simulink model "Target_Control_System"  (R2021b)
settings: Solver=FixedStepDiscrete  StartTime=0.0  StopTime=5  RelTol=1e-3
PreLoadFcn:
  | RTWConfigurationCB('preloadfcn', bdroot);
PostLoadFcn:
  | load('configuration/data_struct.mat');
  | load('configuration/fluxMaps_propMotor.mat');
  | load('configuration/parameterInit_PROP.mat');
  | load('configuration/parameterInit_PUMP.mat');
  | load('configuration/parameterInit_PITCH.mat');
  | load('configuration/parameterInit_TILT.mat');
  | %load('configuration/base_workspace_signal_definition.mat');
  | %load('resolvedatastores_to_baseworkspace_for_faster_simulation.mat');
model workspace (MAT data in the model file):
  SIMULATION_OPTIONS : Simulink.Parameter (value not decoded)
  TARGET_CODE_GEN : Simulink.Parameter (value not decoded)
  TCS_SAMPLE_FREQ_HZ : Simulink.Parameter (value not decoded)
symbols that are objects in the model workspace (value not decoded): TARGET_CODE_GEN, TCS_SAMPLE_FREQ_HZ
undefined symbols (not defined in the file): A_DQ_REF_LPF_INIT__PITCH, A_DQ_REF_LPF_INIT__PROP, A_DQ_REF_LPF_INIT__PUMP, A_DQ_REF_LPF_INIT__TILT, A_OBSERVER_CONFIDENCE_INIT__PITCH, A_OBSERVER_CONFIDENCE_INIT__PROP, A_OBSERVER_CONFIDENCE_INIT__PUMP, A_OBSERVER_CONFIDENCE_INIT__TILT, ACTUATOR_MAX_ANGLE_TRIP__PITCH, ACTUATOR_MIN_ANGLE_TRIP__PITCH, ACTUATOR_POS_SENSOR_INV_DIRECTION__PITCH, ACTUATOR_POS_SENSOR_INV_DIRECTION__TILT, ACTUATOR_POS_SENSOR_OFFSET__PITCH, ACTUATOR_POS_SENSOR_OFFSET__TILT, ADC_scaler1_baseaddr_TILT, ADC_SCALER_FLOAT_TO_FIXPOINT_EXPANSION, ANGLE_ELEC_FROM_SENSOR_OFFSET_INIT__PITCH, ANGLE_ELEC_FROM_SENSOR_OFFSET_INIT__PROP, ANGLE_ELEC_FROM_SENSOR_OFFSET_INIT__PUMP, ANGLE_ELEC_FROM_SENSOR_OFFSET_INIT__TILT, AUTO_CLEAR_FAULTS_ENABLED__PITCH, AUTO_CLEAR_FAULTS_ENABLED__PROP, AUTO_CLEAR_FAULTS_ENABLED__PUMP, AUTO_CLEAR_FAULTS_ENABLED__TILT, AUTO_CLEAR_FAULTS_WAIT_TICKS__PITCH, AUTO_CLEAR_FAULTS_WAIT_TICKS__PROP, AUTO_CLEAR_FAULTS_WAIT_TICKS__PUMP, AUTO_CLEAR_FAULTS_WAIT_TICKS__TILT, AUTO_I_ZERO_IDLE_TICKS__PITCH, AUTO_I_ZERO_IDLE_TICKS__PROP, AUTO_I_ZERO_IDLE_TICKS__PUMP, AUTO_I_ZERO_IDLE_TICKS__TILT, AUTO_I_ZERO_OFFSET_IDC_THRESHOLD__PITCH, AUTO_I_ZERO_OFFSET_IDC_THRESHOLD__PROP, AUTO_I_ZERO_OFFSET_IDC_THRESHOLD__PUMP, AUTO_I_ZERO_OFFSET_IDC_THRESHOLD__TILT, AUTO_I_ZERO_OFFSET_IPH_THRESHOLD__PITCH, AUTO_I_ZERO_OFFSET_IPH_THRESHOLD__PROP, AUTO_I_ZERO_OFFSET_IPH_THRESHOLD__PUMP, AUTO_I_ZERO_OFFSET_IPH_THRESHOLD__TILT, AUTO_SENSORLESS_SWITCHOVER_DISABLE_OMEGA, AUTO_SENSORLESS_SWITCHOVER_ENABLE_OMEGA, AUTO_SENSORLESS_SWITCHOVER_MIN_CONFIDENCE, AUXILIARY_PROTECTION_UNIT_BASEADDR__TILT, blanking_max_error_omega_INIT_PITCH, blanking_max_error_omega_INIT_TILT, blanking_max_error_position_INIT_PITCH, blanking_max_error_position_INIT_TILT, BRUTE_START_I_Q_REF_RAMP_SPEED__PITCH, BRUTE_START_I_Q_REF_RAMP_SPEED__PROP, BRUTE_START_I_Q_REF_RAMP_SPEED__PUMP, BRUTE_START_I_Q_REF_RAMP_SPEED__TILT, CONTROL_LOOP_DT_INIT__PITCH, CONTROL_LOOP_DT_INIT__PROP, CONTROL_LOOP_DT_INIT__PUMP, CONTROL_LOOP_DT_INIT__TILT, CORRECTION_FILTER_SCALE__PITCH, CORRECTION_FILTER_SCALE__PROP, CORRECTION_FILTER_SCALE__PUMP, CORRECTION_FILTER_SCALE__TILT ... (+458)
libraries: simulink x178, Reusables_Lib x24
(part 11 of 47)

== system Target_Control_System/Target_Control_System/InterruptFunction/propMotor_isrTask/currentController/Subsystem ==
  Enable : EnablePort
  Abs : Abs
  Abs1 : Abs
  Add1 : Sum
  Data Store Read10 : DataStoreRead  DataStoreName=oProp  DataStoreElements=oProp.oIsr_.oIn_.fFluxFeedforwardGainRampOut_  IndexOptions=Index vector (dialog)  Indices=1  OutputSizes=1
  Data Store Read11 : DataStoreRead  DataStoreName=oProp  DataStoreElements=oProp.oIsr_.oState_.fId_  IndexOptions=Index vector (dialog)  Indices=1  OutputSizes=1
  Data Store Read12 : DataStoreRead  DataStoreName=oProp  DataStoreElements=oProp.oIsr_.oParam_.oPiDataId_.oParameter_.fKp_  IndexOptions=Index vector (dialog)  Indices=1  OutputSizes=1
  Data Store Read13 : DataStoreRead  DataStoreName=oProp  DataStoreElements=oProp.oIsr_.oIn_.fOneOverUdc_  IndexOptions=Index vector (dialog)  Indices=1  OutputSizes=1
  Data Store Read14 : DataStoreRead  DataStoreName=oProp  DataStoreElements=oProp.oIsr_.oIn_.fOneOverUdc_  IndexOptions=Index vector (dialog)  Indices=1  OutputSizes=1
  Data Store Read15 : DataStoreRead  DataStoreName=mdl_prop_fOmegaE  IndexOptions=Index vector (dialog)  Indices=1  OutputSizes=1
  Data Store Read16 : DataStoreRead  DataStoreName=mdl_prop_fOmegaE  IndexOptions=Index vector (dialog)  Indices=1  OutputSizes=1
  Data Store Read17 : DataStoreRead  DataStoreName=oProp  DataStoreElements=oProp.oIsr_.oParam_.fOverspeedProtectionLimitOmegaE_  IndexOptions=Index vector (dialog)  Indices=1  OutputSizes=1
  Data Store Read18 : DataStoreRead  DataStoreName=oProp  DataStoreElements=oProp.oIsr_.oIn_.fIqRefRampOut_  IndexOptions=Index vector (dialog)  Indices=1  OutputSizes=1
  Data Store Read19 : DataStoreRead  DataStoreName=oProp  DataStoreElements=oProp.oIsr_.oState_.fSoftILimitActual_  IndexOptions=Index vector (dialog)  Indices=1  OutputSizes=1
  Data Store Read2 : DataStoreRead  DataStoreName=oProp  DataStoreElements=oProp.oIsr_.oState_.fIq_  IndexOptions=Index vector (dialog)  Indices=1  OutputSizes=1
  Data Store Read24 : DataStoreRead  DataStoreName=oProp  DataStoreElements=oProp.oIsr_.oParam_.oPiDataId_.oParameter_.fLoopDt_  IndexOptions=Index vector (dialog)  Indices=1  OutputSizes=1
  Data Store Read25 : DataStoreRead  DataStoreName=oProp  DataStoreElements=oProp.oIsr_.oParam_.oPiDataId_.oParameter_.fIntMax_  IndexOptions=Index vector (dialog)  Indices=1  OutputSizes=1
  Data Store Read26 : DataStoreRead  DataStoreName=oProp  DataStoreElements=oProp.oIsr_.oParam_.oPiDataId_.oParameter_.fOutMax_  IndexOptions=Index vector (dialog)  Indices=1  OutputSizes=1
  Data Store Read27 : DataStoreRead  DataStoreName=oProp  DataStoreElements=oProp.oIsr_.oParam_.fMaximumVoltageVectorLengthSquared_  IndexOptions=Index vector (dialog)  Indices=1  OutputSizes=1
  Data Store Read28 : DataStoreRead  DataStoreName=oProp  DataStoreElements=oProp.oIsr_.oParam_.oPiDataId_.oParameter_.fIntMin_  IndexOptions=Index vector (dialog)  Indices=1  OutputSizes=1
  Data Store Read29 : DataStoreRead  DataStoreName=oProp  DataStoreElements=oProp.oIsr_.oParam_.oPiDataId_.oParameter_.fOutMin_  IndexOptions=Index vector (dialog)  Indices=1  OutputSizes=1
  Data Store Read3 : DataStoreRead  DataStoreName=oProp  DataStoreElements=oProp.oIsr_.oIn_.fIdRefFractionOfIq_  IndexOptions=Index vector (dialog)  Indices=1  OutputSizes=1
  Data Store Read30 : DataStoreRead  DataStoreName=oProp  DataStoreElements=oProp.oIsr_.oParam_.oPiDataIq_.oParameter_.fKp_  IndexOptions=Index vector (dialog)  Indices=1  OutputSizes=1
  Data Store Read33 : DataStoreRead  DataStoreName=oProp  DataStoreElements=oProp.oIsr_.oParam_.oPiDataIq_.oParameter_.fLoopDt_  IndexOptions=Index vector (dialog)  Indices=1  OutputSizes=1
  Data Store Read34 : DataStoreRead  DataStoreName=oProp  DataStoreElements=oProp.oIsr_.oParam_.oPiDataIq_.oParameter_.fIntMax_  IndexOptions=Index vector (dialog)  Indices=1  OutputSizes=1
  Data Store Read35 : DataStoreRead  DataStoreName=oProp  DataStoreElements=oProp.oIsr_.oParam_.oPiDataIq_.oParameter_.fOutMax_  IndexOptions=Index vector (dialog)  Indices=1  OutputSizes=1
  Data Store Read36 : DataStoreRead  DataStoreName=oProp  DataStoreElements=oProp.oIsr_.oParam_.oPiDataIq_.oParameter_.fIntMin_  IndexOptions=Index vector (dialog)  Indices=1  OutputSizes=1
  Data Store Read37 : DataStoreRead  DataStoreName=oProp  DataStoreElements=oProp.oIsr_.oParam_.oPiDataIq_.oParameter_.fOutMin_  IndexOptions=Index vector (dialog)  Indices=1  OutputSizes=1
  Data Store Read4 : DataStoreRead  DataStoreName=oProp  DataStoreElements=oProp.oIsr_.oIn_.fIdRefRampOut_  IndexOptions=Index vector (dialog)  Indices=1  OutputSizes=1
  Data Store Read40 : DataStoreRead  DataStoreName=oProp  DataStoreElements=oProp.oIsr_.oParam_.oPiDataIq_.oParameter_.fKi_  IndexOptions=Index vector (dialog)  Indices=1  OutputSizes=1
  Data Store Read5 : DataStoreRead  DataStoreName=oProp  DataStoreElements=oProp.oIsr_.oParam_.oPiDataId_.fState_  IndexOptions=Index vector (dialog)  Indices=1  OutputSizes=1
  Data Store Read6 : DataStoreRead  DataStoreName=oProp  DataStoreElements=oProp.oIsr_.oIn_.fOneOverUdc_  IndexOptions=Index vector (dialog)  Indices=1  OutputSizes=1
  Data Store Read7 : DataStoreRead  DataStoreName=oProp  DataStoreElements=oProp.oIsr_.oParam_.oPiDataId_.oParameter_.fKi_  IndexOptions=Index vector (dialog)  Indices=1  OutputSizes=1
  Data Store Read8 : DataStoreRead  DataStoreName=oProp  DataStoreElements=oProp.oIsr_.oParam_.oPiDataIq_.fState_  IndexOptions=Index vector (dialog)  Indices=1  OutputSizes=1
  Data Store Read9 : DataStoreRead  DataStoreName=oProp  DataStoreElements=oProp.oIsr_.oState_.fFluxMainMagnitudeLpf_  IndexOptions=Index vector (dialog)  Indices=1  OutputSizes=1
  Data Store Write1 : DataStoreWrite  DataStoreName=oProp  DataStoreElements=oProp.oIsr_.oState_.fUqRefPiContrib_  IndexOptions=Index vector (dialog)  Indices=1  OutputSizes=1
  Data Store Write2 : DataStoreWrite  DataStoreName=oProp  DataStoreElements=oProp.oIsr_.oState_.fUdRef_  IndexOptions=Index vector (dialog)  Indices=1  OutputSizes=1
  Data Store Write3 : DataStoreWrite  DataStoreName=oProp  DataStoreElements=oProp.oIsr_.oState_.fUqRef_  IndexOptions=Index vector (dialog)  Indices=1  OutputSizes=1
  Data Store Write31 : DataStoreWrite  DataStoreName=oProp  DataStoreElements=oProp.oIsr_.oParam_.oPiDataId_.fState_  IndexOptions=Index vector (dialog)  Indices=1  OutputSizes=1
  Data Store Write8 : DataStoreWrite  DataStoreName=oProp  DataStoreElements=oProp.oIsr_.oParam_.oPiDataIq_.fState_  IndexOptions=Index vector (dialog)  Indices=1  OutputSizes=1
  Divide1 : Product  Inputs=**
  Equal : RelationalOperator  Operator=>  OutDataTypeStr=boolean  RndMeth=Simplest
  Equal3 : RelationalOperator  Operator=<  OutDataTypeStr=boolean  RndMeth=Simplest
  Flux Feed-forward : Subsystem
  Limit Voltage Vector : Subsystem
  NOT : Logic  Operator=NOT  AllPortsSameDT=off  OutDataTypeStr=boolean
  PI Id Current Controller : Subsystem
  PI Iq Current Controller : Subsystem
  Product : Product
  Product1 : Product
  Sign : Signum
  Subsystem : Subsystem
  Subsystem1 : Subsystem
  Switch : Switch  Criteria=u2 > Threshold
  Switch1 : Switch  Criteria=u2 > Threshold
  wires:
  Subsystem1/1(Output) -> Switch1/3
  Subsystem/1(Output) -> Switch1/1
  Switch1/1 -> Product1/2  "fOverspeedProtectionScaler_"
  Switch/1 -> Product1/1  "fTemp"
  Sign/1 -> Product/1
  Product/1 -> Switch/1
  Equal3/1 -> Switch/2
  Data Store Read19/1 -> Equal3/1, Product/2
  Abs1/1 -> Equal3/2
  Data Store Read18/1 -> Abs1/1, Switch/3, Sign/1
  NOT/1 -> Subsystem1/Enable
  Equal/1 -> Subsystem/Enable, NOT/1, Switch1/2
  Data Store Read17/1 -> Equal/2
  Abs/1 -> Equal/1
  Data Store Read15/1 -> Abs/1
  Add1/1 -> PI Id Current Controller/2(fTarget)
  Data Store Read4/1 -> Add1/1
  Data Store Read10/1 -> Flux Feed-forward/3(fFluxFeedforwardGainRampOut)
  Divide1/1 -> Add1/2
  Data Store Read13/1 -> Flux Feed-forward/4(fOneOverUdc)
  Flux Feed-forward/1(fUqRef) -> Limit Voltage Vector/3(fUqRef)
  Data Store Read27/1 -> Limit Voltage Vector/2(fMaximumVoltageVectorLengthSquared)
  Data Store Read16/1 -> Flux Feed-forward/5(mdl_tilt_fOmegaE)
  Limit Voltage Vector/1(fUdRef_out) -> Data Store Write2/1
  PI Id Current Controller/1(fOutput) -> Limit Voltage Vector/1(fUdRef)
  Data Store Read3/1 -> Divide1/1
  Product1/1 -> PI Iq Current Controller/2(fTarget), Divide1/2
  Data Store Read9/1 -> Flux Feed-forward/2(fFluxMainMagnitudeLpf)
  Limit Voltage Vector/2(fUqRef_out) -> Data Store Write3/1
  PI Iq Current Controller/1(fOutput) -> Flux Feed-forward/1(fUqRefPiContrib), Data Store Write1/1
  Data Store Read36/1 -> PI Iq Current Controller/9(fIntMin)
  PI Id Current Controller/2(*fpState) -> Data Store Write31/1
  Data Store Read34/1 -> PI Iq Current Controller/7(fIntMax)
  Data Store Read8/1 -> PI Iq Current Controller/11(fState)
  Data Store Read12/1 -> PI Id Current Controller/3(fKp)
  Data Store Read26/1 -> PI Id Current Controller/8(fOutMax)
  Data Store Read40/1 -> PI Iq Current Controller/4(fKi)
  PI Iq Current Controller/2(*fpState) -> Data Store Write8/1
  Data Store Read35/1 -> PI Iq Current Controller/8(fOutMax)
  Data Store Read14/1 -> PI Id Current Controller/5(fScale)
  Data Store Read30/1 -> PI Iq Current Controller/3(fKp)
  Data Store Read5/1 -> PI Id Current Controller/11(fState)
  Data Store Read37/1 -> PI Iq Current Controller/10(fOutMin)
  Data Store Read7/1 -> PI Id Current Controller/4(fKi)
  Data Store Read2/1 -> PI Iq Current Controller/1(fActual)
  Data Store Read33/1 -> PI Iq Current Controller/6(fLoopDt)
  Data Store Read6/1 -> PI Iq Current Controller/5(fScale)
  Data Store Read11/1 -> PI Id Current Controller/1(fActual)
  Data Store Read29/1 -> PI Id Current Controller/10(fOutMin)
  Data Store Read24/1 -> PI Id Current Controller/6(fLoopDt)
  Data Store Read25/1 -> PI Id Current Controller/7(fIntMax)
  Data Store Read28/1 -> PI Id Current Controller/9(fIntMin)

== system Target_Control_System/Target_Control_System/InterruptFunction/propMotor_isrTask/fluxAngleCalculation/Angle Clip ==
  Angle_In : Inport
  Add1 : Sum  Inputs=-+
  Add12 : Sum  Inputs=-+
  Add2 : Sum
  Add3 : Sum
  Equal1 : RelationalOperator  Operator=>  OutDataTypeStr=boolean  RndMeth=Simplest
  Equal2 : RelationalOperator  Operator=<  OutDataTypeStr=boolean  RndMeth=Simplest
  Equal3 : RelationalOperator  Operator=<  OutDataTypeStr=boolean  RndMeth=Simplest
  Equal5 : RelationalOperator  Operator=>  OutDataTypeStr=boolean  RndMeth=Simplest
  Pi : Constant  Value=pi  OutDataTypeStr=single  SampleTime=-1
  Pi1 : Constant  Value=2*pi  OutDataTypeStr=single  SampleTime=-1
  Pi2 : Constant  Value=-pi  OutDataTypeStr=single  SampleTime=-1
  Pi3 : Constant  Value=2*pi  OutDataTypeStr=single  SampleTime=-1
  Pi4 : Constant  Value=-pi  OutDataTypeStr=single  SampleTime=-1
  Pi8 : Constant  Value=pi  OutDataTypeStr=single  SampleTime=-1
  Switch{1..3,5} (4 alike) : Switch  Criteria=u2 > Threshold  Threshold=0.5
  Angle_Out : Outport
  wires:
  Switch3/1 -> Switch2/1
  Equal2/1 -> Switch3/2
  Switch5/1 -> Switch2/3, Add3/2, Equal3/1
  Add2/1 -> Switch3/1
  Pi3/1 -> Add3/1, Add2/1
  Add3/1 -> Switch3/3, Equal2/1, Add2/2
  Pi4/1 -> Equal2/2
  Switch2/1 -> Angle_Out/1
  Equal3/1 -> Switch2/2
  Pi2/1 -> Equal3/2
  Switch1/1 -> Switch5/1
  Add1/1 -> Switch1/1
  Equal5/1 -> Switch1/2
  Pi8/1 -> Equal5/2
  Add12/1 -> Equal5/1, Add1/2, Switch1/3
  Pi/1 -> Equal1/2
  Equal1/1 -> Switch5/2
  Angle_In/1 -> Add12/2, Equal1/1, Switch5/3
  Pi1/1 -> Add12/1, Add1/1

== system Target_Control_System/Target_Control_System/InterruptFunction/propMotor_isrTask/fluxAngleCalculation/ModelSource ==
  note: 1) Add Subsystem or Model blocks as valid variant choices.
      | 2) You cannot connect blocks at this level. At simulation, connectivity is automatically
      | determined, based on the active variant and port name matching.
  DoNotIncludeCustomCode : Subsystem  TreatAsAtomicUnit=on  VariantControl=TARGET_CODE_GEN == 0
  IncludeCustomCode : Subsystem  TreatAsAtomicUnit=on  VariantControl=(default)

== system Target_Control_System/Target_Control_System/InterruptFunction/propMotor_isrTask/fluxAngleCalculation/Subsystem ==
  Enable : EnablePort
  Data Store Read66 : DataStoreRead  DataStoreName=oProp  DataStoreElements=oProp.oIsr_.oIn_.fOmegaERefRampOut_  IndexOptions=Index vector (dialog)  Indices=1  OutputSizes=1
  Integrator with Angle Wrapper : Subsystem
  Integrator with Angle Wrapper_OLD : Subsystem  Commented=on
  Angle : Outport
  wires:
  Integrator with Angle Wrapper/1(Angle) -> Angle/1
  Data Store Read66/1 -> Integrator with Angle Wrapper/1(Omega)

== system Target_Control_System/Target_Control_System/InterruptFunction/propMotor_isrTask/fluxAngleCalculation/Subsystem1 ==
  In1 : Inport
  In2 : Inport  Port=2
  Enable : EnablePort
  Add1 : Sum
  Angle Clip : Subsystem
  Angle_Out : Outport
  wires:
  Add1/1 -> Angle Clip/1(Angle_In)
  In2/1 -> Add1/2
  In1/1 -> Add1/1
  Angle Clip/1(Angle_Out) -> Angle_Out/1

== system Target_Control_System/Target_Control_System/InterruptFunction/propMotor_isrTask/fluxAngleCalculation/vsincos()1 ==
  fFluxMasterAngle : Inport
  fFluxMasterAngleBdwd : Inport  Port=2
  Enable : EnablePort
  Cos2 : Trigonometry  Operator=cos
  Cos3 : Trigonometry  Operator=cos
  Data Store Write1 : DataStoreWrite  DataStoreName=mdl_fFluxMasterAngle_cos_  IndexOptions=Index vector (dialog)  Indices=1  OutputSizes=1
  Data Store Write2 : DataStoreWrite  DataStoreName=mdl_fFluxMasterAngle_sin_  IndexOptions=Index vector (dialog)  Indices=1  OutputSizes=1
  Data Store Write7 : DataStoreWrite  DataStoreName=mdl_fFluxMasterAngleBkwd_sin_  IndexOptions=Index vector (dialog)  Indices=1  OutputSizes=1
  Data Store Write8 : DataStoreWrite  DataStoreName=mdl_fFluxMasterAngleBkwd_cos_  IndexOptions=Index vector (dialog)  Indices=1  OutputSizes=1
  Sin2 : Trigonometry
  Sin3 : Trigonometry
  wires:
  fFluxMasterAngle/1 -> Sin2/1, Cos2/1
  fFluxMasterAngleBdwd/1 -> Sin3/1, Cos3/1
  Sin2/1 -> Data Store Write2/1
  Cos2/1 -> Data Store Write1/1
  Sin3/1 -> Data Store Write7/1
  Cos3/1 -> Data Store Write8/1

== system Target_Control_System/Target_Control_System/InterruptFunction/propMotor_isrTask/fluxObserver/piControllerStep_fOmegaE1 ==
  fActual : Inport
  fTarget : Inport  Port=2
  fKp : Inport  Port=3
  fKi : Inport  Port=4
  fScale : Inport  Port=5
  fLoopDt : Inport  Port=6
  fIntMax : Inport  Port=7
  fOutMax : Inport  Port=8
  fIntMin : Inport  Port=9
  fOutMin : Inport  Port=10
  fState : Inport  Port=11
  Add : Sum  Inputs=|++
  Mux : Mux  Inputs=3
  Mux1 : Mux  Inputs=3
  Product : Product
  Saturation Dynamic : simulink/Discontinuities/Saturation Dynamic  OutMin=[]  OutMax=[]  OutDataTypeStr=Inherit: Same as second input  OutDataType=fixdt(1, 16)  OutScaling=2^-10  DoSatur=off
  Saturation Dynamic1 : simulink/Discontinuities/Saturation Dynamic  OutMin=[]  OutMax=[]  OutDataTypeStr=Inherit: Same as second input  OutDataType=fixdt(1, 16)  OutScaling=2^-10  DoSatur=off
  Scope3 : Scope  NumInputPorts=6
  Sum1 : Sum  Inputs=++|
  Sum22 : Sum  Inputs=-+|
  fError * fKi_ * fScale : Fcn  Expr=u(1)*u(2)*u(3)
  fError * fKp_ * fScale1 : Fcn  Expr=u(1)*u(2)*u(3)
  fOutput : Outport
  *fpState : Outport  Port=2
  wires:
  fLoopDt/1 -> Product/2
  fOutMax/1 -> Saturation Dynamic1/1
  fOutMin/1 -> Saturation Dynamic1/3
  fIntMin/1 -> Saturation Dynamic/3
  fIntMax/1 -> Saturation Dynamic/1
  Add/1 -> Saturation Dynamic/2
  fState/1 -> Add/2
  Product/1 -> Add/1
  Mux1/1 -> fError * fKp_ * fScale1/1
  fKi/1 -> Mux/2
  fScale/1 -> Mux/1, Mux1/3
  fKp/1 -> Mux1/2
  Mux/1 -> fError * fKi_ * fScale/1
  Saturation Dynamic1/1 -> fOutput/1, Scope3/6
  Sum1/1 -> Saturation Dynamic1/2  "fError"
  fError * fKp_ * fScale1/1 -> Sum1/1, Scope3/4
  Saturation Dynamic/1 -> Scope3/5, *fpState/1, Sum1/2  "*fpState"
  fActual/1 -> Sum22/1, Scope3/2
  fTarget/1 -> Sum22/2, Scope3/1
  fError * fKi_ * fScale/1 -> Product/1
  Sum22/1 -> Scope3/3, Mux/3, Mux1/1  "fError"

== system Target_Control_System/Target_Control_System/InterruptFunction/propMotor_isrTask/pwmGeneration/Subsystem ==
  note: // moved here, originating from main layer
      | // Ramp soft current limit back up to the setpoint (it is reduced in the main interrupt loop)
  Enable : EnablePort
  Constant1 : Constant  OutDataTypeStr=int32  SampleTime=-1
  Constant11 : Constant  Value=-1  SampleTime=-1
  Constant12 : Constant  Value=-1  SampleTime=-1
  Constant13 : Constant  Value=-1  SampleTime=-1
  Constant2 : Constant  Value=0.5  OutDataTypeStr=single  SampleTime=-1
  Constant4 : Constant  Value=0.5  OutDataTypeStr=single  SampleTime=-1
  Constant6 : Constant  Value=0.5  OutDataTypeStr=single  SampleTime=-1
  Data Store Read1 : DataStoreRead  DataStoreName=mdl_fFluxMasterAngleBkwd_cos_  IndexOptions=Index vector (dialog)  Indices=1  OutputSizes=1
  Data Store Read10 : DataStoreRead  DataStoreName=oProp  DataStoreElements=oProp.oIsr_.oParam_.fMaximumDuty_  IndexOptions=Index vector (dialog)  Indices=1  OutputSizes=1
  Data Store Read11 : DataStoreRead  DataStoreName=oProp  DataStoreElements=oProp.oIsr_.oParam_.fMaximumDuty_  IndexOptions=Index vector (dialog)  Indices=1  OutputSizes=1
  Data Store Read12 : DataStoreRead  DataStoreName=oProp  DataStoreElements=oProp.oIsr_.oState_.fSoftILimitActual_  IndexOptions=Index vector (dialog)  Indices=1  OutputSizes=1
  Data Store Read13 : DataStoreRead  DataStoreName=mdl_fFluxMasterAngleBkwd_sin_  IndexOptions=Index vector (dialog)  Indices=1  OutputSizes=1
  Data Store Read14 : DataStoreRead  DataStoreName=oProp  DataStoreElements=oProp.oIsr_.oParam_.fSoftILimitA_  IndexOptions=Index vector (dialog)  Indices=1  OutputSizes=1
  Data Store Read18 : DataStoreRead  DataStoreName=oProp  DataStoreElements=oProp.oIsr_.oParam_.fHalfPositiveDuty_  IndexOptions=Index vector (dialog)  Indices=1  OutputSizes=1
  Data Store Read19 : DataStoreRead  DataStoreName=oProp  DataStoreElements=oProp.oIsr_.oParam_.iInverseDirection_  IndexOptions=Index vector (dialog)  Indices=1  OutputSizes=1
  Data Store Read2 : DataStoreRead  DataStoreName=oProp  DataStoreElements=oProp.oIsr_.oState_.fUdRef_  IndexOptions=Index vector (dialog)  Indices=1  OutputSizes=1
  Data Store Read3 : DataStoreRead  DataStoreName=oProp  DataStoreElements=oProp.oIsr_.oState_.fUqRef_  IndexOptions=Index vector (dialog)  Indices=1  OutputSizes=1
  Data Store Read4 : DataStoreRead  DataStoreName=oProp  DataStoreElements=oProp.oIsr_.oParam_.fHalfPositiveDuty_  IndexOptions=Index vector (dialog)  Indices=1  OutputSizes=1
  Data Store Read5 : DataStoreRead  DataStoreName=oProp  DataStoreElements=oProp.oIsr_.oParam_.fHalfPositiveDuty_  IndexOptions=Index vector (dialog)  Indices=1  OutputSizes=1
  Data Store Read6 : DataStoreRead  DataStoreName=oProp  DataStoreElements=oProp.oIsr_.oParam_.fPwmPeriodTicksFloat_  IndexOptions=Index vector (dialog)  Indices=1  OutputSizes=1
  Data Store Read7 : DataStoreRead  DataStoreName=oProp  DataStoreElements=oProp.oIsr_.oParam_.fPwmPeriodTicksFloat_  IndexOptions=Index vector (dialog)  Indices=1  OutputSizes=1
  Data Store Read8 : DataStoreRead  DataStoreName=oProp  DataStoreElements=oProp.oIsr_.oParam_.fPwmPeriodTicksFloat_  IndexOptions=Index vector (dialog)  Indices=1  OutputSizes=1
  Data Store Read9 : DataStoreRead  DataStoreName=oProp  DataStoreElements=oProp.oIsr_.oParam_.fMaximumDuty_  IndexOptions=Index vector (dialog)  Indices=1  OutputSizes=1
  Data Store Write2 : DataStoreWrite  DataStoreName=oProp  DataStoreElements=oProp.oIsr_.oOut_.uiPwmDutyTicksB_  IndexOptions=Index vector (dialog)  Indices=1  OutputSizes=1
  Data Store Write27 : DataStoreWrite  DataStoreName=oProp  DataStoreElements=oProp.oIsr_.oState_.iPwmUpdated_  IndexOptions=Index vector (dialog)  Indices=1  OutputSizes=1
  Data Store Write3 : DataStoreWrite  DataStoreName=oProp  DataStoreElements=oProp.oIsr_.oOut_.uiPwmDutyTicksC_  IndexOptions=Index vector (dialog)  Indices=1  OutputSizes=1
  Data Store Write5 : DataStoreWrite  DataStoreName=oProp  DataStoreElements=oProp.oIsr_.oOut_.uiPwmDutyTicksA_  IndexOptions=Index vector (dialog)  Indices=1  OutputSizes=1
  Data Type Conversion : DataTypeConversion  OutDataTypeStr=uint32
  Data Type Conversion1 : DataTypeConversion  OutDataTypeStr=uint32
  Data Type Conversion2 : DataTypeConversion  OutDataTypeStr=uint32
  Demux : Demux  Outputs=3
  Equal : RelationalOperator  Operator=~=  OutDataTypeStr=boolean  RndMeth=Simplest
  Gain4 : Gain  Gain=0.5
  Max : MinMax  Function=max  Inputs=3
  Max1 : MinMax  Inputs=3
  Mux : Mux  Inputs=2
  Mux5 : Mux
  Product{1,6..10} (6 alike) : Product
  Saturation Dynamic : simulink/Discontinuities/Saturation Dynamic  OutMin=[]  OutMax=[]  OutDataTypeStr=Inherit: Same as second input  OutDataType=fixdt(1, 16)  OutScaling=2^-10  DoSatur=off
  Saturation Dynamic1 : simulink/Discontinuities/Saturation Dynamic  OutMin=[]  OutMax=[]  OutDataTypeStr=Inherit: Same as second input  OutDataType=fixdt(1, 16)  OutScaling=2^-10  DoSatur=off
  Saturation Dynamic2 : simulink/Discontinuities/Saturation Dynamic  OutMin=[]  OutMax=[]  OutDataTypeStr=Inherit: Same as second input  OutDataType=fixdt(1, 16)  OutScaling=2^-10  DoSatur=off
  Subsystem : Subsystem
  Sum1 : Sum  Inputs=|++  OutDataTypeStr=single
  Sum4 : Sum  Inputs=|++  OutDataTypeStr=single
  Sum5 : Sum  Inputs=|++  OutDataTypeStr=single
  Sum6 : Sum  OutDataTypeStr=single
  Sum7 : Sum  Inputs=|+-  OutDataTypeStr=single
  Sum8 : Sum  Inputs=|+-  OutDataTypeStr=single
  Sum9 : Sum  Inputs=|+-  OutDataTypeStr=single
  Switch1 : Switch  Criteria=u2 > Threshold
  alpha/beta to abc1 : Gain  Gain="[1  0; -0.5 sqrt(3)/2; -0.5 -sqrt(3)/2]"  Multiplication=Matrix(K*u) (u vector)
  alpha/beta to abc_inverseDirection1 : Gain  Gain="[1  0; -0.5 -sqrt(3)/2; -0.5 sqrt(3)/2]"  Multiplication=Matrix(K*u) (u vector)
  fUAlphaRef_ = afOutArray[3]*fUdRef - afOutArray[2]*fUqRef : Fcn  Expr=u(4)*u(1)-u(3)*u(2)
  fUBetaRef_ = afOutArray[3]*fUqRef + afOutArray[2]*fUdRef : Fcn  Expr=u(4)*u(2)+u(3)*u(1)
  wires:
  Constant1/1 -> Data Store Write27/1
  Equal/1 -> Subsystem/Enable
  Data Store Read14/1 -> Equal/2
  Data Store Read12/1 -> Equal/1
  alpha/beta to abc_inverseDirection1/1 -> Switch1/1
  Demux/3 -> Sum9/1, Max1/3, Max/3
  Data Store Read9/1 -> Saturation Dynamic/1
  Constant4/1 -> Sum4/2
  Mux5/1 -> fUAlphaRef_ = afOutArray[3]*fUdRef - afOutArray[2]*fUqRef/1, fUBetaRef_ = afOutArray[3]*fUqRef + afOutArray[2]*fUdRef/1
  Data Store Read8/1 -> Product10/2
  Sum6/1 -> Gain4/1  "Umax+Umin"
  Product1/1 -> Sum1/1
  Data Type Conversion/1 -> Data Store Write5/1
  Constant2/1 -> Sum1/2
  Constant6/1 -> Sum5/2
  Data Store Read2/1 -> Mux5/1
  Data Store Read13/1 -> Mux5/3
  Gain4/1 -> Sum9/2, Sum7/2, Sum8/2
  Sum5/1 -> Product10/1
  Sum4/1 -> Product9/1
  Product8/1 -> Data Type Conversion/1
  Data Store Read3/1 -> Mux5/2
  Product10/1 -> Data Type Conversion2/1
  Saturation Dynamic1/1 -> Product6/1
  Mux/1 -> alpha/beta to abc_inverseDirection1/1, alpha/beta to abc1/1
  alpha/beta to abc1/1 -> Switch1/3
  Data Store Read6/1 -> Product8/2
  Demux/1 -> Max1/2, Max/1, Sum7/1
  Max/1 -> Sum6/1
  Constant11/1 -> Saturation Dynamic/3
  Sum7/1 -> Saturation Dynamic/2  "fUaRef"
  Sum8/1 -> Saturation Dynamic1/2  "fUbRef"
  Data Store Read7/1 -> Product9/2
  Data Store Read18/1 -> Product1/2
  Max1/1 -> Sum6/2
  Data Store Read5/1 -> Product7/2
  Product6/1 -> Sum4/1
  Saturation Dynamic/1 -> Product1/1
  Product9/1 -> Data Type Conversion1/1
  Data Store Read4/1 -> Product6/2
  Data Type Conversion2/1 -> Data Store Write3/1
  Demux/2 -> Max1/1, Max/2, Sum8/1
  Data Type Conversion1/1 -> Data Store Write2/1
  Sum1/1 -> Product8/1
  Sum9/1 -> Saturation Dynamic2/2  "fUcRef"
  Constant13/1 -> Saturation Dynamic2/3
  Data Store Read11/1 -> Saturation Dynamic2/1
  Switch1/1 -> Demux/1
  Data Store Read1/1 -> Mux5/4
  fUAlphaRef_ = afOutArray[3]*fUdRef - afOutArray[2]*fUqRef/1 -> Mux/1  "fUAlphaRef_"
  Constant12/1 -> Saturation Dynamic1/3
  Data Store Read19/1 -> Switch1/2
  Saturation Dynamic2/1 -> Product7/1
  fUBetaRef_ = afOutArray[3]*fUqRef + afOutArray[2]*fUdRef/1 -> Mux/2  "fUBetaRef_"
  Data Store Read10/1 -> Saturation Dynamic1/1
  Product7/1 -> Sum5/1

== system Target_Control_System/Target_Control_System/InterruptFunction/propMotor_isrTask/softCurrentLimiting/Subsystem ==
  note: // Some current exceeds the soft current limiter
  fMaxOvershoot : Inport
  Enable : EnablePort
  Abs : Abs
  Add : Sum  Inputs=-+
  Add1 : Sum  Inputs=+-
  Constant : Constant  Value=0  OutDataTypeStr=single  SampleTime=-1
  Constant1 : Constant  Value=0  OutDataTypeStr=single  SampleTime=-1
  Data Store Read1 : DataStoreRead  DataStoreName=oProp  DataStoreElements=oProp.oIsr_.oParam_.fSoftILimitKp_  IndexOptions=Index vector (dialog)  Indices=1  OutputSizes=1
  Data Store Read7 : DataStoreRead  DataStoreName=oProp  DataStoreElements=oProp.oIsr_.oIn_.fIqRefRampOut_  IndexOptions=Index vector (dialog)  Indices=1  OutputSizes=1
  Data Store Read8 : DataStoreRead  DataStoreName=oProp  DataStoreElements=oProp.oIsr_.oState_.fSoftILimitActual_  IndexOptions=Index vector (dialog)  Indices=1  OutputSizes=1
  Data Store Write10 : DataStoreWrite  DataStoreName=oProp  DataStoreElements=oProp.oIsr_.oState_.fSoftILimitActual_  IndexOptions=Index vector (dialog)  Indices=1  OutputSizes=1
  Equal1 : RelationalOperator  Operator=<  OutDataTypeStr=boolean  RndMeth=Simplest
  Equal3 : RelationalOperator  Operator=<  OutDataTypeStr=boolean  RndMeth=Simplest
  Product : Product
  Switch : Switch  Criteria=u2 > Threshold
  Switch1 : Switch  Criteria=u2 > Threshold
  wires:
  Constant1/1 -> Switch1/1
  Switch1/1 -> Data Store Write10/1
  Equal1/1 -> Switch1/2
  Constant/1 -> Equal1/2
  Add1/1 -> Switch/3
  Data Store Read1/1 -> Product/1
  fMaxOvershoot/1 -> Product/2
  Product/1 -> Add/1, Add1/2
  Add/1 -> Switch/1
  Switch/1 -> Equal1/1, Switch1/3
  Equal3/1 -> Switch/2
  Abs/1 -> Equal3/1, Add/2
  Data Store Read7/1 -> Abs/1
  Data Store Read8/1 -> Equal3/2, Add1/1

== system Target_Control_System/Target_Control_System/InterruptFunction/propMotor_setPwm/ModelSourceFPGAProp/DoNotIncludeCustomCode ==

== system Target_Control_System/Target_Control_System/InterruptFunction/propMotor_setPwm/ModelSourceFPGAProp/IncludeCustomCode ==
  System Update : Subsystem  mask(System Update){ShowInLibBrowser=0}
      mask prompts: ShowInLibBrowser "Simulink:masks:CustCodeMaskParam1_MP"
      settings: CopyFcn=cccopyfcn(gcb)  OpenFcn=ccopenfcn('System Update Function')
      mask Help: eval('feval(''rtwprivate'',''rtwhelpview'',''rtw_sys_update_block'')');
      mask DialogControl ShowInLibBrowser Prompt: Mask Parameter 1:
      mask Display: disp('System\nUpdate');

== system Target_Control_System/Target_Control_System/InterruptFunction/pumpMotor_isrTask/abcToAlphaBeta/Integrator with Angle Wrapper ==
  Omega : Inport
  Add : Sum  Commented=on  Inputs=+-
  Add1 : Sum  Commented=on
  Add5 : Sum
  Add6 : Sum  Inputs=+-
  Add7 : Sum
  Constant1 : Constant  Commented=on  Value=2*pi  OutDataTypeStr=single  SampleTime=-1
  Constant11 : Constant  Commented=on  Value=-pi  OutDataTypeStr=single  SampleTime=-1
  Constant12 : Constant  Value=pi  OutDataTypeStr=single  SampleTime=-1
  Constant13 : Constant  Value=-pi  OutDataTypeStr=single  SampleTime=-1
  Constant14 : Constant  Value=2*pi  OutDataTypeStr=single  SampleTime=-1
  Constant15 : Constant  Value=2*pi  OutDataTypeStr=single  SampleTime=-1
  Constant2 : Constant  Commented=on  Value=2*pi  OutDataTypeStr=single  SampleTime=-1
  Constant6 : Constant  Commented=on  Value=pi  OutDataTypeStr=single  SampleTime=-1
  Data Store Read1 : DataStoreRead  DataStoreName=oPump  DataStoreElements=oPump.oIsr_.oParam_.fControlLoopDt_  IndexOptions=Index vector (dialog)  Indices=1  OutputSizes=1
  Data Store Read29 : DataStoreRead  Commented=on  DataStoreName=oProp  DataStoreElements=oProp.oIsr_.oParam_.fControlLoopDt_  IndexOptions=Index vector (dialog)  Indices=1  OutputSizes=1
  Discrete-Time Integrator4 : DiscreteIntegrator  Commented=on  IntegratorMethod=Accumulation: Forward Euler  ExternalReset=rising  InitialConditionSource=external  SampleTime=-1  ShowStatePort=on  ICPrevOutput=DiscIntNeverNeededParam  ICPrevScaledInput=DiscIntNeverNeededParam
  Equal3 : RelationalOperator  Commented=on  Operator=>  OutDataTypeStr=boolean  RndMeth=Simplest
  Equal4 : RelationalOperator  Commented=on  Operator=<  OutDataTypeStr=boolean  RndMeth=Simplest
  Equal5 : RelationalOperator  Operator=>  OutDataTypeStr=boolean  RndMeth=Simplest
  Equal6 : RelationalOperator  Operator=<  OutDataTypeStr=boolean  RndMeth=Simplest
  Logical Operator : Logic  Commented=on  Operator=OR  AllPortsSameDT=off  OutDataTypeStr=boolean
  Logical Operator2 : Logic  Operator=OR  AllPortsSameDT=off  OutDataTypeStr=boolean
  Product1 : Product
  Product16 : Product  Commented=on
  Switch1 : Switch  Commented=on  Criteria=u2 > Threshold  Threshold=0.5
  Switch2 : Switch  Commented=on  Criteria=u2 > Threshold  Threshold=0.5
  Switch5 : Switch  Criteria=u2 > Threshold
  Switch6 : Switch  Criteria=u2 > Threshold  Threshold=0.5
  Switch7 : Switch  Criteria=u2 > Threshold  Threshold=0.5
  Unit Delay1 : UnitDelay  SampleTime=-1  HasFrameUpgradeWarning=on
  Angle : Outport
  wires:
  Switch6/1 -> Switch7/3
  Omega/1 -> Product1/1
  Switch7/1 -> Switch5/1
  Add5/1 -> Switch5/3, Equal5/1, Equal6/1, Add7/1, Add6/1, Switch6/3
  Constant12/1 -> Equal5/2
  Logical Operator2/1 -> Switch5/2
  Unit Delay1/1 -> Add5/1
  Constant15/1 -> Add7/2
  Equal6/1 -> Switch7/2, Logical Operator2/2
  Add6/1 -> Switch6/1
  Product1/1 -> Add5/2
  Data Store Read1/1 -> Product1/2
  Add7/1 -> Switch7/1
  Equal5/1 -> Switch6/2, Logical Operator2/1
  Switch5/1 -> Unit Delay1/1, Angle/1
  Constant13/1 -> Equal6/2
  Constant14/1 -> Add6/2
  Data Store Read29/1 -> Product16/2
  Add/1 -> Switch2/1
  Switch2/1 -> Switch1/3
  Add1/1 -> Switch1/1
  Constant2/1 -> Add1/2
  Constant1/1 -> Add/2
  Equal3/1 -> Switch2/2, Logical Operator/1
  Switch1/1 -> Discrete-Time Integrator4/3
  Constant11/1 -> Equal4/2
  Logical Operator/1 -> Discrete-Time Integrator4/2
  Constant6/1 -> Equal3/2
  Product16/1 -> Discrete-Time Integrator4/1
  Equal4/1 -> Switch1/2, Logical Operator/2
  Discrete-Time Integrator4/State -> Add1/1, Equal4/1, Add/1, Switch2/3, Equal3/1

== system Target_Control_System/Target_Control_System/InterruptFunction/pumpMotor_isrTask/abcToAlphaBeta/Integrator with Angle Wrapper_OLD ==
  Omega : Inport
  Add : Sum  Inputs=+-
  Add1 : Sum
  Constant1 : Constant  Value=2*pi  OutDataTypeStr=single  SampleTime=-1
  Constant11 : Constant  Value=-pi  OutDataTypeStr=single  SampleTime=-1
  Constant2 : Constant  Value=2*pi  OutDataTypeStr=single  SampleTime=-1
  Constant6 : Constant  Value=pi  OutDataTypeStr=single  SampleTime=-1
  Data Store Read29 : DataStoreRead  DataStoreName=oPump  DataStoreElements=oPump.oIsr_.oParam_.fControlLoopDt_  IndexOptions=Index vector (dialog)  Indices=1  OutputSizes=1
  Discrete-Time Integrator4 : DiscreteIntegrator  IntegratorMethod=Accumulation: Forward Euler  ExternalReset=rising  InitialConditionSource=external  SampleTime=-1  ShowStatePort=on  ICPrevOutput=DiscIntNeverNeededParam  ICPrevScaledInput=DiscIntNeverNeededParam
  Equal3 : RelationalOperator  Operator=>  OutDataTypeStr=boolean  RndMeth=Simplest
  Equal4 : RelationalOperator  Operator=<  OutDataTypeStr=boolean  RndMeth=Simplest
  Logical Operator : Logic  Operator=OR  AllPortsSameDT=off  OutDataTypeStr=boolean
  Product16 : Product
  Switch1 : Switch  Criteria=u2 > Threshold  Threshold=0.5
  Switch2 : Switch  Criteria=u2 > Threshold  Threshold=0.5
  Angle : Outport
  wires:
  Omega/1 -> Product16/1
  Data Store Read29/1 -> Product16/2
  Add/1 -> Switch2/1
  Switch2/1 -> Switch1/3
  Add1/1 -> Switch1/1
  Constant2/1 -> Add1/2
  Constant1/1 -> Add/2
  Equal3/1 -> Switch2/2, Logical Operator/1
  Switch1/1 -> Discrete-Time Integrator4/3
  Constant11/1 -> Equal4/2
  Discrete-Time Integrator4/1 -> Angle/1
  Logical Operator/1 -> Discrete-Time Integrator4/2
  Constant6/1 -> Equal3/2
  Product16/1 -> Discrete-Time Integrator4/1
  Equal4/1 -> Switch1/2, Logical Operator/2
  Discrete-Time Integrator4/State -> Add1/1, Equal4/1, Add/1, Switch2/3, Equal3/1

== system Target_Control_System/Target_Control_System/InterruptFunction/pumpMotor_isrTask/abcToAlphaBeta/ModelSource ==
  note: 1) Add Subsystem or Model blocks as valid variant choices.
      | 2) You cannot connect blocks at this level. At simulation, connectivity is automatically
      | determined, based on the active variant and port name matching.
  DoNotIncludeCustomCode : Subsystem  TreatAsAtomicUnit=on  VariantControl=TARGET_CODE_GEN == 0
  IncludeCustomCode : Subsystem  TreatAsAtomicUnit=on  VariantControl=(default)

== system Target_Control_System/Target_Control_System/InterruptFunction/pumpMotor_isrTask/abcToAlphaBeta/vsincos()1 ==
  Input : Inport
  Input1 : Inport  Port=2
  Enable : EnablePort
  Cos : Trigonometry  Operator=cos
  Cos1 : Trigonometry  Operator=cos
  Data Store Write : DataStoreWrite  DataStoreName=mdl_pump_fUphFilterDelayAngleRad_cos_  IndexOptions=Index vector (dialog)  Indices=1  OutputSizes=1
  Data Store Write10 : DataStoreWrite  DataStoreName=mdl_pump_fFluxMainAngleRaw2_sin_  IndexOptions=Index vector (dialog)  Indices=1  OutputSizes=1
  Data Store Write11 : DataStoreWrite  DataStoreName=mdl_pump_fFluxMainAngleRaw2_cos_  IndexOptions=Index vector (dialog)  Indices=1  OutputSizes=1
  Data Store Write6 : DataStoreWrite  DataStoreName=mdl_pump_fUphFilterDelayAngleRad_sin_  IndexOptions=Index vector (dialog)  Indices=1  OutputSizes=1
  Sin : Trigonometry
  Sin1 : Trigonometry
  wires:
  Input/1 -> Sin/1, Cos/1
  Cos/1 -> Data Store Write/1
  Input1/1 -> Sin1/1, Cos1/1
  Sin1/1 -> Data Store Write10/1
  Sin/1 -> Data Store Write6/1
  Cos1/1 -> Data Store Write11/1

== system Target_Control_System/Target_Control_System/InterruptFunction/pumpMotor_isrTask/currentController/Subsystem ==
  Enable : EnablePort
  Abs : Abs
  Abs1 : Abs
  Add1 : Sum
  Data Store Read1 : DataStoreRead  DataStoreName=oPump  DataStoreElements=oPump.oIsr_.oParam_.oPiDataIq_.oParameter_.fKp_  IndexOptions=Index vector (dialog)  Indices=1  OutputSizes=1
  Data Store Read10 : DataStoreRead  DataStoreName=oPump  DataStoreElements=oPump.oIsr_.oParam_.oPiDataIq_.oParameter_.fOutMin_  IndexOptions=Index vector (dialog)  Indices=1  OutputSizes=1
  Data Store Read11 : DataStoreRead  DataStoreName=oPump  DataStoreElements=oPump.oIsr_.oState_.fId_  IndexOptions=Index vector (dialog)  Indices=1  OutputSizes=1
  Data Store Read12 : DataStoreRead  DataStoreName=oPump  DataStoreElements=oPump.oIsr_.oParam_.oPiDataId_.oParameter_.fKp_  IndexOptions=Index vector (dialog)  Indices=1  OutputSizes=1
  Data Store Read13 : DataStoreRead  DataStoreName=oPump  DataStoreElements=oPump.oIsr_.oParam_.oPiDataIq_.fState_  IndexOptions=Index vector (dialog)  Indices=1  OutputSizes=1
  Data Store Read14 : DataStoreRead  DataStoreName=oPump  DataStoreElements=oPump.oIsr_.oIn_.fOneOverUdc_  IndexOptions=Index vector (dialog)  Indices=1  OutputSizes=1
  Data Store Read15 : DataStoreRead  DataStoreName=oPump  DataStoreElements=oPump.oIsr_.oParam_.oPiDataIq_.oParameter_.fKi_  IndexOptions=Index vector (dialog)  Indices=1  OutputSizes=1
  Data Store Read16 : DataStoreRead  DataStoreName=mdl_pump_fOmegaE  IndexOptions=Index vector (dialog)  Indices=1  OutputSizes=1
  Data Store Read17 : DataStoreRead  DataStoreName=oPump  DataStoreElements=oPump.oIsr_.oIn_.fFluxFeedforwardGainRampOut_  IndexOptions=Index vector (dialog)  Indices=1  OutputSizes=1
  Data Store Read18 : DataStoreRead  DataStoreName=oPump  DataStoreElements=oPump.oIsr_.oIn_.fOneOverUdc_  IndexOptions=Index vector (dialog)  Indices=1  OutputSizes=1
  Data Store Read19 : DataStoreRead  DataStoreName=mdl_pump_fOmegaE  IndexOptions=Index vector (dialog)  Indices=1  OutputSizes=1
  Data Store Read2 : DataStoreRead  DataStoreName=oPump  DataStoreElements=oPump.oIsr_.oState_.fIq_  IndexOptions=Index vector (dialog)  Indices=1  OutputSizes=1
  Data Store Read20 : DataStoreRead  DataStoreName=oPump  DataStoreElements=oPump.oIsr_.oIn_.fIdRefFractionOfIq_  IndexOptions=Index vector (dialog)  Indices=1  OutputSizes=1
  Data Store Read21 : DataStoreRead  DataStoreName=oPump  DataStoreElements=oPump.oIsr_.oIn_.fIdRefRampOut_  IndexOptions=Index vector (dialog)  Indices=1  OutputSizes=1
  Data Store Read22 : DataStoreRead  DataStoreName=oPump  DataStoreElements=oPump.oIsr_.oState_.fFluxMainMagnitudeLpf_  IndexOptions=Index vector (dialog)  Indices=1  OutputSizes=1
  Data Store Read23 : DataStoreRead  DataStoreName=oPump  DataStoreElements=oPump.oIsr_.oParam_.fOverspeedProtectionLimitOmegaE_  IndexOptions=Index vector (dialog)  Indices=1  OutputSizes=1
  Data Store Read24 : DataStoreRead  DataStoreName=oPump  DataStoreElements=oPump.oIsr_.oParam_.oPiDataId_.oParameter_.fLoopDt_  IndexOptions=Index vector (dialog)  Indices=1  OutputSizes=1
  Data Store Read25 : DataStoreRead  DataStoreName=oPump  DataStoreElements=oPump.oIsr_.oParam_.oPiDataId_.oParameter_.fIntMax_  IndexOptions=Index vector (dialog)  Indices=1  OutputSizes=1
  Data Store Read26 : DataStoreRead  DataStoreName=oPump  DataStoreElements=oPump.oIsr_.oParam_.oPiDataId_.oParameter_.fOutMax_  IndexOptions=Index vector (dialog)  Indices=1  OutputSizes=1
  Data Store Read27 : DataStoreRead  DataStoreName=oPump  DataStoreElements=oPump.oIsr_.oParam_.fMaximumVoltageVectorLengthSquared_  IndexOptions=Index vector (dialog)  Indices=1  OutputSizes=1
  Data Store Read28 : DataStoreRead  DataStoreName=oPump  DataStoreElements=oPump.oIsr_.oParam_.oPiDataId_.oParameter_.fIntMin_  IndexOptions=Index vector (dialog)  Indices=1  OutputSizes=1
  Data Store Read29 : DataStoreRead  DataStoreName=oPump  DataStoreElements=oPump.oIsr_.oParam_.oPiDataId_.oParameter_.fOutMin_  IndexOptions=Index vector (dialog)  Indices=1  OutputSizes=1
  Data Store Read3 : DataStoreRead  DataStoreName=oPump  DataStoreElements=oPump.oIsr_.oParam_.oPiDataId_.fState_  IndexOptions=Index vector (dialog)  Indices=1  OutputSizes=1
  Data Store Read30 : DataStoreRead  DataStoreName=oPump  DataStoreElements=oPump.oIsr_.oIn_.fIqRefRampOut_  IndexOptions=Index vector (dialog)  Indices=1  OutputSizes=1
  Data Store Read31 : DataStoreRead  DataStoreName=oPump  DataStoreElements=oPump.oIsr_.oState_.fSoftILimitActual_  IndexOptions=Index vector (dialog)  Indices=1  OutputSizes=1
  Data Store Read4 : DataStoreRead  DataStoreName=oPump  DataStoreElements=oPump.oIsr_.oIn_.fOneOverUdc_  IndexOptions=Index vector (dialog)  Indices=1  OutputSizes=1
  Data Store Read5 : DataStoreRead  DataStoreName=oPump  DataStoreElements=oPump.oIsr_.oParam_.oPiDataIq_.oParameter_.fLoopDt_  IndexOptions=Index vector (dialog)  Indices=1  OutputSizes=1
  Data Store Read6 : DataStoreRead  DataStoreName=oPump  DataStoreElements=oPump.oIsr_.oParam_.oPiDataIq_.oParameter_.fIntMax_  IndexOptions=Index vector (dialog)  Indices=1  OutputSizes=1
  Data Store Read7 : DataStoreRead  DataStoreName=oPump  DataStoreElements=oPump.oIsr_.oParam_.oPiDataId_.oParameter_.fKi_  IndexOptions=Index vector (dialog)  Indices=1  OutputSizes=1
  Data Store Read8 : DataStoreRead  DataStoreName=oPump  DataStoreElements=oPump.oIsr_.oParam_.oPiDataIq_.oParameter_.fOutMax_  IndexOptions=Index vector (dialog)  Indices=1  OutputSizes=1
  Data Store Read9 : DataStoreRead  DataStoreName=oPump  DataStoreElements=oPump.oIsr_.oParam_.oPiDataIq_.oParameter_.fIntMin_  IndexOptions=Index vector (dialog)  Indices=1  OutputSizes=1
  Data Store Write31 : DataStoreWrite  DataStoreName=oPump  DataStoreElements=oPump.oIsr_.oParam_.oPiDataId_.fState_  IndexOptions=Index vector (dialog)  Indices=1  OutputSizes=1
  Data Store Write4 : DataStoreWrite  DataStoreName=oPump  DataStoreElements=oPump.oIsr_.oState_.fUqRefPiContrib_  IndexOptions=Index vector (dialog)  Indices=1  OutputSizes=1
  Data Store Write5 : DataStoreWrite  DataStoreName=oPump  DataStoreElements=oPump.oIsr_.oState_.fUdRef_  IndexOptions=Index vector (dialog)  Indices=1  OutputSizes=1
  Data Store Write7 : DataStoreWrite  DataStoreName=oPump  DataStoreElements=oPump.oIsr_.oState_.fUqRef_  IndexOptions=Index vector (dialog)  Indices=1  OutputSizes=1
  Data Store Write8 : DataStoreWrite  DataStoreName=oPump  DataStoreElements=oPump.oIsr_.oParam_.oPiDataIq_.fState_  IndexOptions=Index vector (dialog)  Indices=1  OutputSizes=1
  Divide1 : Product  Inputs=**
  Equal : RelationalOperator  Operator=>  OutDataTypeStr=boolean  RndMeth=Simplest
  Equal3 : RelationalOperator  Operator=<  OutDataTypeStr=boolean  RndMeth=Simplest
  Flux Feed-forward : Subsystem
  Limit Voltage Vector : Subsystem
  NOT : Logic  Operator=NOT  AllPortsSameDT=off  OutDataTypeStr=boolean
  PI Id Current Controller : Subsystem
  PI Iq Current Controller : Subsystem
  Product : Product
  Product1 : Product
  Sign : Signum
  Subsystem : Subsystem
  Subsystem1 : Subsystem
  Switch : Switch  Criteria=u2 > Threshold
  Switch1 : Switch  Criteria=u2 > Threshold
  wires:
  Data Store Read30/1 -> Abs1/1, Switch/3, Sign/1
  Abs1/1 -> Equal3/2
  Data Store Read31/1 -> Equal3/1, Product/2
  Data Store Read16/1 -> Abs/1
  Switch1/1 -> Product1/2  "fOverspeedProtectionScaler_"
  Equal3/1 -> Switch/2
  Subsystem/1(Output) -> Switch1/1
  Abs/1 -> Equal/1
  Sign/1 -> Product/1
  Switch/1 -> Product1/1  "fTemp"
  NOT/1 -> Subsystem1/Enable
  Equal/1 -> Subsystem/Enable, NOT/1, Switch1/2
  Subsystem1/1(Output) -> Switch1/3
  Product/1 -> Switch/1
  Data Store Read23/1 -> Equal/2
  Flux Feed-forward/1(fUqRef) -> Limit Voltage Vector/3(fUqRef)
  PI Id Current Controller/1(fOutput) -> Limit Voltage Vector/1(fUdRef)
  Limit Voltage Vector/1(fUdRef_out) -> Data Store Write5/1
  Data Store Read19/1 -> Flux Feed-forward/5(mdl_pump_fOmegaE)
  Data Store Read21/1 -> Add1/1
  PI Iq Current Controller/1(fOutput) -> Flux Feed-forward/1(fUqRefPiContrib), Data Store Write4/1
  Data Store Read27/1 -> Limit Voltage Vector/2(fMaximumVoltageVectorLengthSquared)
  Data Store Read20/1 -> Divide1/1
  Limit Voltage Vector/2(fUqRef_out) -> Data Store Write7/1
  Data Store Read22/1 -> Flux Feed-forward/2(fFluxMainMagnitudeLpf)
  Data Store Read18/1 -> Flux Feed-forward/4(fOneOverUdc)
  Divide1/1 -> Add1/2
  Data Store Read17/1 -> Flux Feed-forward/3(fFluxFeedforwardGainRampOut)
  Product1/1 -> Divide1/2, PI Iq Current Controller/2(fTarget)
  Data Store Read5/1 -> PI Iq Current Controller/6(fLoopDt)
  Data Store Read9/1 -> PI Iq Current Controller/9(fIntMin)
  Data Store Read15/1 -> PI Iq Current Controller/4(fKi)
  PI Iq Current Controller/2(*fpState) -> Data Store Write8/1
  Data Store Read2/1 -> PI Iq Current Controller/1(fActual)
  Data Store Read26/1 -> PI Id Current Controller/8(fOutMax)
  PI Id Current Controller/2(*fpState) -> Data Store Write31/1
  Data Store Read12/1 -> PI Id Current Controller/3(fKp)
  Data Store Read4/1 -> PI Iq Current Controller/5(fScale)
  Data Store Read11/1 -> PI Id Current Controller/1(fActual)
  Data Store Read7/1 -> PI Id Current Controller/4(fKi)
  Data Store Read6/1 -> PI Iq Current Controller/7(fIntMax)
  Data Store Read25/1 -> PI Id Current Controller/7(fIntMax)
  Data Store Read13/1 -> PI Iq Current Controller/11(fState)
  Add1/1 -> PI Id Current Controller/2(fTarget)
  Data Store Read1/1 -> PI Iq Current Controller/3(fKp)
  Data Store Read14/1 -> PI Id Current Controller/5(fScale)
  Data Store Read10/1 -> PI Iq Current Controller/10(fOutMin)
  Data Store Read24/1 -> PI Id Current Controller/6(fLoopDt)
  Data Store Read28/1 -> PI Id Current Controller/9(fIntMin)
  Data Store Read29/1 -> PI Id Current Controller/10(fOutMin)
  Data Store Read8/1 -> PI Iq Current Controller/8(fOutMax)
  Data Store Read3/1 -> PI Id Current Controller/11(fState)

== system Target_Control_System/Target_Control_System/InterruptFunction/pumpMotor_isrTask/fluxAngleCalculations/Angle Clip1 ==
  Angle_In : Inport
  Add1 : Sum  Inputs=-+
  Add12 : Sum  Inputs=-+
  Add2 : Sum
  Add3 : Sum
  Equal1 : RelationalOperator  Operator=>  OutDataTypeStr=boolean  RndMeth=Simplest
  Equal2 : RelationalOperator  Operator=<  OutDataTypeStr=boolean  RndMeth=Simplest
  Equal3 : RelationalOperator  Operator=<  OutDataTypeStr=boolean  RndMeth=Simplest
  Equal5 : RelationalOperator  Operator=>  OutDataTypeStr=boolean  RndMeth=Simplest
  Pi : Constant  Value=pi  OutDataTypeStr=single  SampleTime=-1
  Pi1 : Constant  Value=2*pi  OutDataTypeStr=single  SampleTime=-1
  Pi2 : Constant  Value=-pi  OutDataTypeStr=single  SampleTime=-1
  Pi3 : Constant  Value=2*pi  OutDataTypeStr=single  SampleTime=-1
  Pi4 : Constant  Value=-pi  OutDataTypeStr=single  SampleTime=-1
  Pi8 : Constant  Value=pi  OutDataTypeStr=single  SampleTime=-1
  Switch{1..3,5} (4 alike) : Switch  Criteria=u2 > Threshold  Threshold=0.5
  Angle_Out : Outport
  wires:
  Switch3/1 -> Switch2/1
  Equal2/1 -> Switch3/2
  Switch5/1 -> Switch2/3, Add3/2, Equal3/1
  Add2/1 -> Switch3/1
  Pi3/1 -> Add3/1, Add2/1
  Add3/1 -> Switch3/3, Equal2/1, Add2/2
  Pi4/1 -> Equal2/2
  Switch2/1 -> Angle_Out/1
  Equal3/1 -> Switch2/2
  Pi2/1 -> Equal3/2
  Switch1/1 -> Switch5/1
  Add1/1 -> Switch1/1
  Equal5/1 -> Switch1/2
  Pi8/1 -> Equal5/2
  Add12/1 -> Equal5/1, Add1/2, Switch1/3
  Pi/1 -> Equal1/2
  Equal1/1 -> Switch5/2
  Angle_In/1 -> Add12/2, Equal1/1, Switch5/3
  Pi1/1 -> Add12/1, Add1/1

== system Target_Control_System/Target_Control_System/InterruptFunction/pumpMotor_isrTask/fluxAngleCalculations/ModelSource1 ==
  note: 1) Add Subsystem or Model blocks as valid variant choices.
      | 2) You cannot connect blocks at this level. At simulation, connectivity is automatically
      | determined, based on the active variant and port name matching.
  DoNotIncludeCustomCode : Subsystem  TreatAsAtomicUnit=on  VariantControl=TARGET_CODE_GEN == 0
  IncludeCustomCode : Subsystem  TreatAsAtomicUnit=on  VariantControl=(default)

== system Target_Control_System/Target_Control_System/InterruptFunction/pumpMotor_isrTask/fluxAngleCalculations/Subsystem2 ==
  Enable : EnablePort
  Data Store Read66 : DataStoreRead  DataStoreName=oPump  DataStoreElements=oPump.oIsr_.oIn_.fOmegaERefRampOut_  IndexOptions=Index vector (dialog)  Indices=1  OutputSizes=1
  Integrator with Angle Wrapper : Subsystem
  Integrator with Angle Wrapper_OLD : Subsystem
  Angle : Outport
  wires:
  Integrator with Angle Wrapper/1(Angle) -> Angle/1
  Data Store Read66/1 -> Integrator with Angle Wrapper/1(Omega)

== system Target_Control_System/Target_Control_System/InterruptFunction/pumpMotor_isrTask/fluxAngleCalculations/Subsystem3 ==
  In1 : Inport
  In2 : Inport  Port=2
  Enable : EnablePort
  Add1 : Sum
  Angle Clip : Subsystem
  Angle_Out : Outport
  wires:
  Add1/1 -> Angle Clip/1(Angle_In)
  In2/1 -> Add1/2
  In1/1 -> Add1/1
  Angle Clip/1(Angle_Out) -> Angle_Out/1
